simulink model "regulator_LQR_discrete"  (R2023a)
settings: Solver=ode45  StartTime=0.0  StopTime=3  RelTol=1e-3  EnableMultiTasking=on
values from neighbouring files (symbols this model uses):
  B_tilda = [sysdis.B(1) Bw_bar(1,1) Bw_bar(1,2); sysdis.B(2) Bw_bar(2,1) Bw_bar(2,2)]    [motor.m]
  D_tilda = [0 0 0 ; 0 0 0]    [motor.m]
  sysdis = c2d(sys,Ts)    [motor.m]
  Ts = 0.001    [parameters.m]
  u_max = 12    [constraints.m]
  u_min = 0    [constraints.m]
  uBar = -(A(1,1)*(-A(2,2)*nref/A(2,1)) + A(1,2)*nref)*L    [motor.m]
  w = [1 1]'    [parameters.m]
  x0 = [0.2 70.3]'    [motor.m]
  yref = [iref nref]'    [motor.m]
undefined symbols (not defined in the file or in its folder): Kd
settings Model: Creator=Administrator  LastModifiedBy=teora
settings SolverCC: AlgebraicLoopSolver=TrustRegion
settings DataIOCC: LimitDataPoints=on  SaveFormat=Array  SignalLoggingSaveFormat=ModelDataLogs  ReturnWorkspaceOutputs=off
settings OptimizationCC: ReuseModelBlockBuffer=off  ExpressionDepthLimit=2147483647  InitFltsAndDblsToZero=on  LifeSpan=inf
settings DebuggingCC: UnderspecifiedInitializationDetection=Classic  MergeDetectMultiDrivingBlocksExec=none  SolverPrmCheckMsg=warning  FcnCallInpInsideContextMsg=warning  UnconnectedInputMsg=warning  UnconnectedOutputMsg=warning  UnconnectedLineMsg=warning  StateNameClashWarn=warning  SFUnexpectedBacktrackingDiag=warning  SFNoUnconditionalDefaultTransitionDiag=warning  SFExecutionAtInitializationDiag=none  ArithmeticOperatorsInVariantConditions=warning
settings HardwareCC: ProdBitPerPointer=32  ProdBitPerSizeT=32  ProdBitPerPtrDiffT=32  ProdLargestAtomicFloat=None  ProdIntDivRoundTo=Undefined  ProdEndianess=Unspecified  ProdWordSize=32  ProdHWDeviceType=32-bit Generic
settings ModelReferenceCC: EnableRefExpFcnMdlSchedulingChecks=on  PropagateSignalLabelsOutOfModel=off
settings SFSimCC: SimUseLocalCustomCode=off  CustomCodeUndefinedFunction=UseInterfaceOnly
settings RTWCC: RTWUseLocalCustomCode=off  DLArmComputeVersion=19.05
settings CodeAppCC: StateflowObjectComments=on
settings GRTTargetCC: TargetLangStandard=C89/C90 (ANSI)  CombineOutputUpdateFcns=off  GRTInterface=on
settings ConfigComp: CovMetricSettings=dw  CovSaveCumulativeToWorkspaceVar=on  CovSaveSingleToWorkspaceVar=on  CovExternalEMLEnable=off  CovSFcnEnable=off

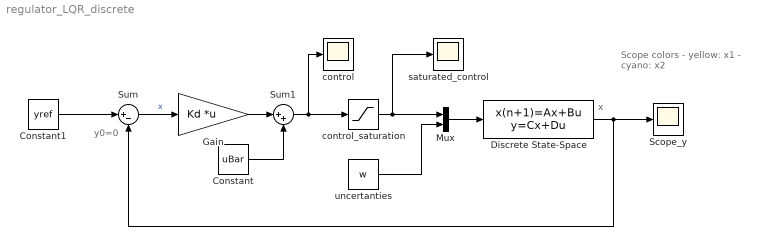
== system regulator_LQR_discrete ==
  note: y0=0
  note: x
  note: Scope colors
      | - yellow: x1
      | - cyano: x2
  Constant : Constant  Value=uBar
  Constant1 : Constant  Value=yref
  Discrete State-Space : DiscreteStateSpace  A=sysdis.A  B=B_tilda  C=sysdis.C  D=D_tilda  InitialCondition=x0  SampleTime=Ts
  Gain : Gain  Gain=Kd  Multiplication=Matrix(K*u)
  Mux : Mux  Inputs=2
  Scope_y : Scope
  Sum : Sum  Inputs=|+-
  Sum1 : Sum  Inputs=|++
  control : Scope
  control_saturation : Saturate  UpperLimit=u_max  LowerLimit=u_min
  saturated_control : Scope
  uncertanties : Constant  Value=w
  wires:
  control_saturation/1 -> Mux/1, saturated_control/1
  Sum/1 -> Gain/1  "x"
  Discrete State-Space/1 -> Scope_y/1, Sum/2
  Constant1/1 -> Sum/1
  Mux/1 -> Discrete State-Space/1
  uncertanties/1 -> Mux/2
  Sum1/1 -> control/1, control_saturation/1
  Gain/1 -> Sum1/1
  Constant/1 -> Sum1/2
